simulink model "SpdDemSwt_DD"  (R2016b)
settings: configuration reference "CodeGenConfigSet" (kept outside this file)
values from neighbouring files (symbols this model uses):
  SpdDemSwt_tiDebHiLo_C = Calibration.Parameter    [init_SpdDemSwt_DD.m]
  SpdDemSwt_tiDebLoHi_C = Calibration.Parameter    [init_SpdDemSwt_DD.m]
undefined symbols (not defined in the file or in its folder): SpdDemSwt_DD_DT
libraries: CXLib x1
settings Model: Creator=lenovo  LastModifiedBy=xuxingpei
settings ConfigSetRef: SourceLocation=Base Workspace

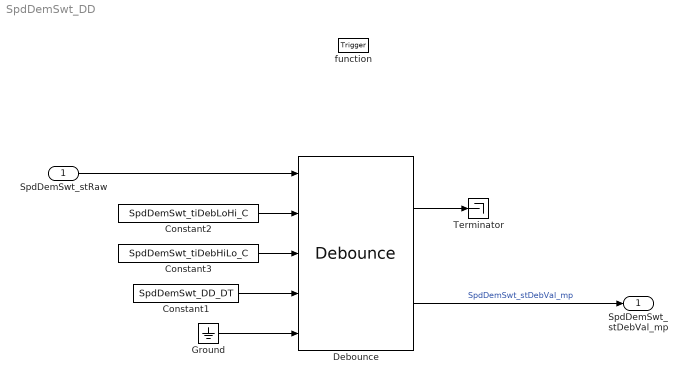
== system SpdDemSwt_DD ==
  SpdDemSwt_stRaw : Inport  Description=speed demand switch raw value from hardware pin  OutMin=0  OutMax=1  OutDataTypeStr=boolean
  function : TriggerPort  TriggerType=function-call  VariantControl=Variant
  Constant1 : Constant  Value=SpdDemSwt_DD_DT
  Constant2 : Constant  Value=SpdDemSwt_tiDebLoHi_C
  Constant3 : Constant  Value=SpdDemSwt_tiDebHiLo_C
  Debounce : CXLib/Debounce
  Ground : Ground
  Terminator : Terminator
  SpdDemSwt_stDebVal_mp : Outport  Description=Debounced speed demand switch status  OutMin=0  OutMax=1  OutDataTypeStr=boolean
  wires:
  Debounce/1 -> Terminator/1
  Debounce/2 -> SpdDemSwt_stDebVal_mp/1  "SpdDemSwt_stDebVal_mp"
  Ground/1 -> Debounce/5
  Constant1/1 -> Debounce/4
  Constant3/1 -> Debounce/3
  Constant2/1 -> Debounce/2
  SpdDemSwt_stRaw/1 -> Debounce/1
